simulink model "wariant2"  (R2021b)
settings: Solver=VariableStepAuto  StartTime=0.0  StopTime=10.0  RelTol=1e-3
values from neighbouring files (symbols this model uses):
  A_2 = transpose(A_1)    [stp01.m]
  B_2 = transpose(C_1)    [stp01.m]
  start_x = [0 0 0]    [stp01.m]
  Tp = 0.5    [stp01.m]
settings Model: Creator=USER  LastModifiedBy=USER

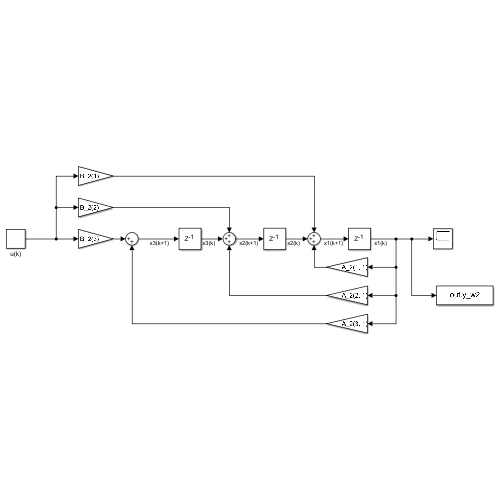
[thumbnail: Simulink's stored preview of the top-level diagram]
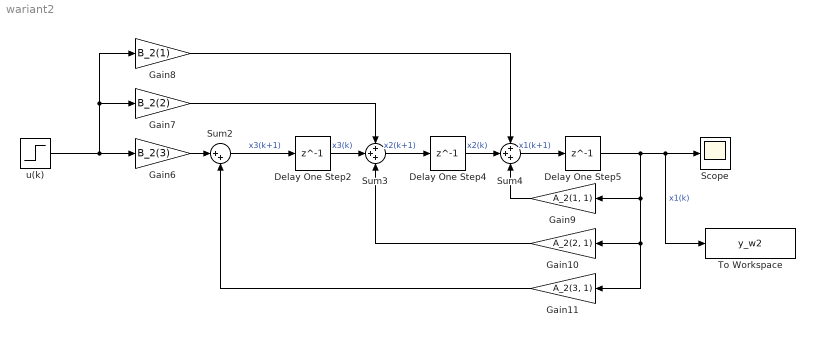
== system wariant2 ==
  Delay One Step2 : Delay  DelayLength=1  InitialCondition=start_x(1)
  Delay One Step4 : Delay  DelayLength=1  InitialCondition=start_x(2)
  Delay One Step5 : Delay  DelayLength=1  InitialCondition=start_x(3)
  Gain10 : Gain  Gain=A_2(2, 1)
  Gain11 : Gain  Gain=A_2(3, 1)
  Gain6 : Gain  Gain=B_2(3)
  Gain7 : Gain  Gain=B_2(2)
  Gain8 : Gain  Gain=B_2(1)
  Gain9 : Gain  Gain=A_2(1, 1)
  Scope : Scope
  Sum2 : Sum  Inputs=|++
  Sum3 : Sum  Inputs=+++
  Sum4 : Sum  Inputs=+++
  To Workspace : ToWorkspace  VariableName=y_w2  SaveFormat=Structure With Time  SampleTime=Tp
  u(k) : Step  SampleTime=Tp
  wires:
  Delay One Step4/1 -> Sum4/2  "x2(k)"
  Delay One Step5/1 -> Gain9/1, Gain11/1, Gain10/1, To Workspace/1, Scope/1  "x1(k)"
  Gain8/1 -> Sum4/1
  Sum4/1 -> Delay One Step5/1  "x1(k+1)"
  u(k)/1 -> Gain6/1, Gain7/1, Gain8/1
  Gain10/1 -> Sum3/3
  Sum3/1 -> Delay One Step4/1  "x2(k+1)"
  Delay One Step2/1 -> Sum3/2  "x3(k)"
  Gain6/1 -> Sum2/1
  Gain11/1 -> Sum2/2
  Gain9/1 -> Sum4/3
  Sum2/1 -> Delay One Step2/1  "x3(k+1)"
  Gain7/1 -> Sum3/1
